simulink model "hvac"  (R2021b)
settings: Solver=FixedStepAuto  StartTime=0.0  StopTime=inf  FixedStep=.1  RelTol=1e-3  AbsTol=1e-6
InitFcn:
  | mpath = get_param(bdroot, 'FileName')
  | [path,name,ext]=fileparts(mpath)
  | path
  | addpath(path);
  | load('testData.mat')
StopFcn:
  | if isLogging
  |     outputJson = jsonencode(struct("simTime", output.simTime, "InsideTemp1", simOutput.InsideTemp1, "OutsideTemp1", simOutput.OutsideTemp1, "Heat1", simInput.Heat1, "Cool1", simInput.Cool1, ...
  |         "InsideTemp2", simOutput.InsideTemp2, "OutsideTemp2", simOutput.OutsideTemp2, "Heat2", simInput.Heat2, "Cool2", simInput.Cool2));
  |     fprintf(outputFile, "%s,", outputJson);
  |     fclose(outputFile);
  | end
model workspace (MATLAB code in the model file + MAT data in the model file):
  LWall = 0.2
  LWindow = 0.01
  M = 1778.36911446
  Mdot = 1
  PLC_IP_Address = 'localhost'
  RWall = 1.52148180317e-06
  RWindow = 5.93542260209e-07
  Req = 0.00153711229591
  THeater = 50
  TinIC = 20
  c = 1005.4
  cost = 2.5e-08
  densAir = 1.225
  htHouse = 4
  htWindows = 1
  kWall = 136.8
  kWindow = 2808
  lenHouse = 30
  numWindows = 6
  pitRoof = 0.698131700798
  r2d = 57.2957795131
  wallArea = 960.897659797
  widHouse = 10
  widWindows = 1
  windowArea = 6
  other statements: sldemo_househeat_data
undefined symbols (not defined in the file or in its folder): simInput
libraries: simulink_extras x4
PauseFcn:
  | if exist("fixedStepSize", "var") == 0
  |     fixedStepSize = simOutput.SimulationMetadata.ModelInfo.SolverInfo.FixedStepSize;
  | end
  | output.simTime = simOutput.SimulationMetadata.ModelInfo.StopTime - fixedStepSize;
  | output.InsideTemp1 = simOutput.InsideTemp1;
  | output.OutsideTemp1 = simOutput.OutsideTemp1;
  | output.InsideTemp2 = simOutput.InsideTemp2;
  | output.OutsideTemp2 = simOutput.OutsideTemp2;
ContinueFcn:
  | if isLogging
  |     outputJson = jsonencode(struct("simTime", output.simTime, "InsideTemp1", simOutput.InsideTemp1, "OutsideTemp1", simOutput.OutsideTemp1, "Heat1", simInput.Heat1, "Cool1", simInput.Cool1, ...
  |         "InsideTemp2", simOutput.InsideTemp2, "OutsideTemp2", simOutput.OutsideTemp2, "Heat2", simInput.Heat2, "Cool2", simInput.Cool2));
  |     fprintf(outputFile, "%s,", outputJson);
  | end
Description:
  | Thermal Model of a House
  | 
  | This demo illustrates how you can use Simulink(R) to create the thermal model of
  | a house. This system models the outdoor environment, the thermal
  | characteristics of the house, and the house heating system.
  | 
  | The sldemo_househeat_data.m file initializes data in the model workspace.
  | To make changes, you can edit the model workspace directly or edit the MATLAB(R) file
  | and re-load the model workspace.
  | 
  | To view the model workspace, select View > Model Explorer
  | from the Simulink editor.
  | 
  | Note: Time is given in units of hours
settings Model: PacingRate=100  Creator=The MathWorks, Inc.  LastModifiedBy=CCRE
settings SolverCC: AutoScaleAbsTol=off  AlgebraicLoopSolver=TrustRegion
settings DataIOCC: ExternalInput=[]  InitialState=[]  SaveFormat=Array  SaveOutput=off  SaveTime=off  SignalLoggingName=sldemo_househeat_output  ReturnWorkspaceOutputsName=simOutput
settings OptimizationCC: BlockReduction=off  BooleanDataType=off  ExpressionDepthLimit=2147483647  InitFltsAndDblsToZero=on  LifeSpan=inf  BufferReusableBoundary=off
settings DebuggingCC: SaveWithParameterizedLinksMsg=none  UnderspecifiedInitializationDetection=Classic  MergeDetectMultiDrivingBlocksExec=none  SignalResolutionControl=TryResolveAllWithWarning  MultiTaskDSMMsg=warning  MultiTaskCondExecSysMsg=none  IntegerOverflowMsg=none  FcnCallInpInsideContextMsg=warning  BusObjectLabelMismatch=none  StateNameClashWarn=warning  SFUnexpectedBacktrackingDiag=warning  SFNoUnconditionalDefaultTransitionDiag=warning  SFExecutionAtInitializationDiag=none  SFMachineParentedDataDiag=warning  IntegerSaturationMsg=none  ArithmeticOperatorsInVariantConditions=warning
settings HardwareCC: ProdBitPerPointer=32  ProdBitPerSizeT=32  ProdBitPerPtrDiffT=32  ProdLargestAtomicFloat=None  ProdIntDivRoundTo=Undefined  ProdEndianess=Unspecified  ProdWordSize=32  ProdHWDeviceType=32-bit Generic  TargetBitPerPointer=64  TargetBitPerSizeT=64  TargetBitPerPtrDiffT=64  TargetLongLongMode=on  TargetIntDivRoundTo=Zero  TargetEndianess=LittleEndian  TargetWordSize=64  TargetHWDeviceType=MATLAB Host  ProdEqTarget=off
settings ModelReferenceCC: PropagateSignalLabelsOutOfModel=off
settings SFSimCC: SimUseLocalCustomCode=off  CustomCodeUndefinedFunction=UseInterfaceOnly
settings RTWCC: PackageGeneratedCodeAndArtifacts=on  PackageName=HVAC  RTWUseLocalCustomCode=off
settings CodeAppCC: StateflowObjectComments=on
settings GRTTargetCC: TargetFcnLib=ansi_tfl_tmw.mat  TargetLangStandard=C89/C90 (ANSI)  CombineOutputUpdateFcns=off  GRTInterface=on
settings ConfigComp: CovMetricSettings=dw  CovSaveCumulativeToWorkspaceVar=on  CovSaveSingleToWorkspaceVar=on  CovExternalEMLEnable=off

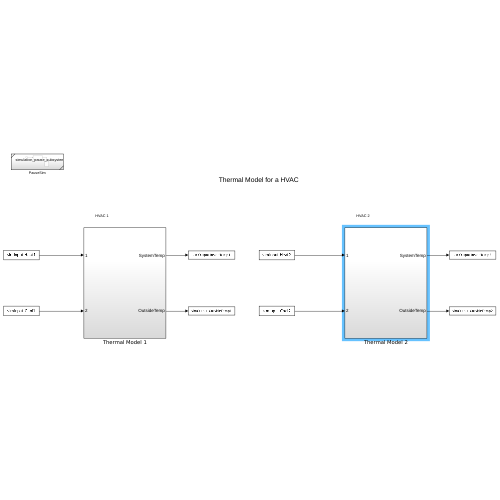
[thumbnail: Simulink's stored preview of the top-level diagram]
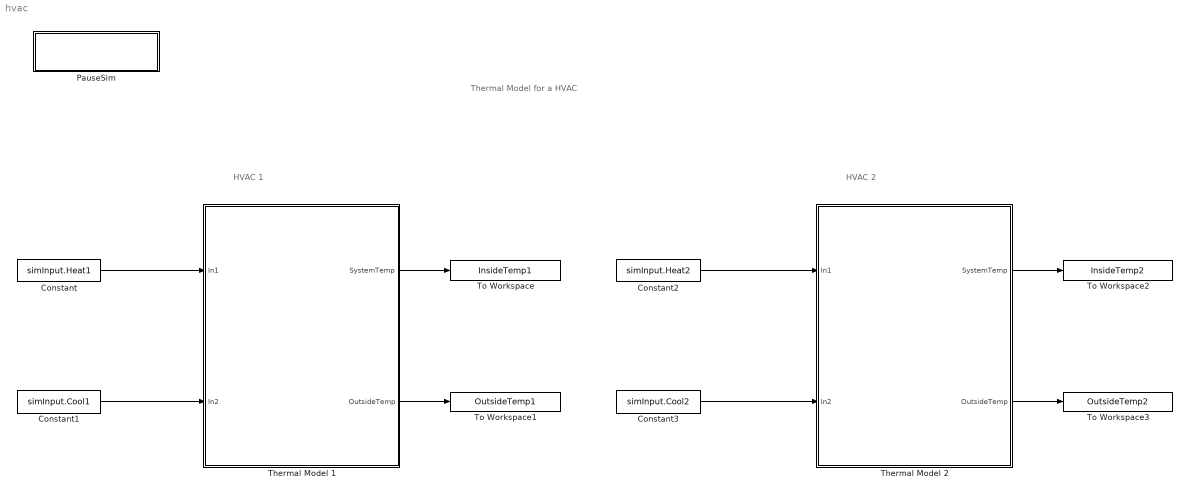
== system hvac ==
  note: HVAC 1
  note: Thermal Model for a HVAC
  note: HVAC 2
  Constant : Constant  Value=simInput.Heat1
  Constant1 : Constant  Value=simInput.Cool1
  Constant2 : Constant  Value=simInput.Heat2
  Constant3 : Constant  Value=simInput.Cool2
  PauseSim : Subsystem  ReferencedSubsystem=simulation_pause_subsystem
  Thermal Model 1 : Subsystem
  Thermal Model 2 : Subsystem
  To Workspace : ToWorkspace  VariableName=InsideTemp1  SampleTime=-1
      settings: MaxDataPoints=1  Save2DSignal=2-D array (concatenate along first dimension)
  To Workspace1 : ToWorkspace  VariableName=OutsideTemp1  SampleTime=-1
      settings: MaxDataPoints=1  Save2DSignal=2-D array (concatenate along first dimension)
  To Workspace2 : ToWorkspace  VariableName=InsideTemp2  SampleTime=-1
      settings: MaxDataPoints=1  Save2DSignal=2-D array (concatenate along first dimension)
  To Workspace3 : ToWorkspace  VariableName=OutsideTemp2  SampleTime=-1
      settings: MaxDataPoints=1  Save2DSignal=2-D array (concatenate along first dimension)
  wires:
  Thermal Model 1/1(SystemTemp) -> To Workspace/1
  Constant1/1 -> Thermal Model 1/2(In2)
  Thermal Model 1/2(OutsideTemp) -> To Workspace1/1
  Constant3/1 -> Thermal Model 2/2(In2)
  Constant/1 -> Thermal Model 1/1(In1)
  Constant2/1 -> Thermal Model 2/1(In1)
  Thermal Model 2/2(OutsideTemp) -> To Workspace3/1
  Thermal Model 2/1(SystemTemp) -> To Workspace2/1

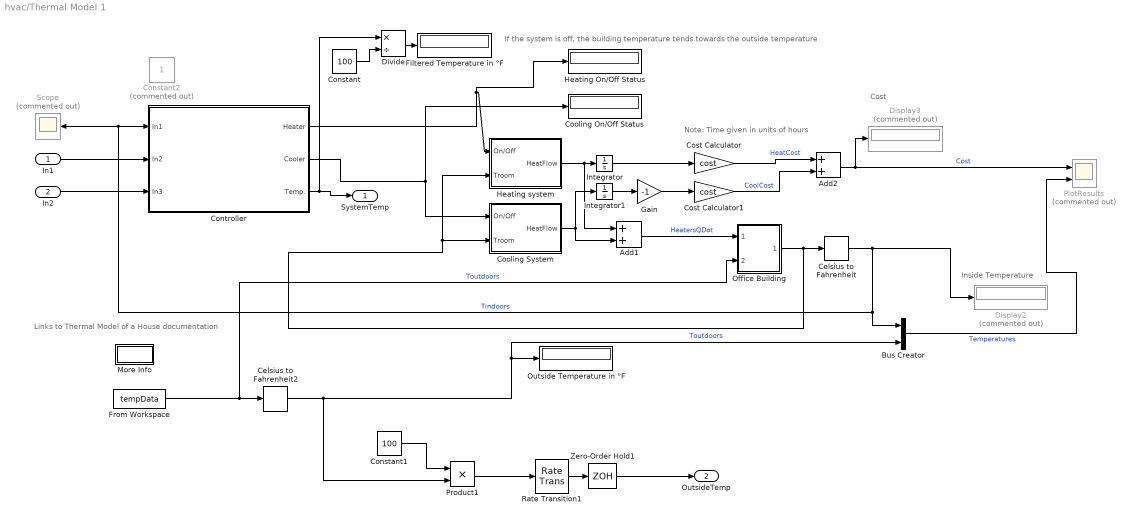
== system hvac/Thermal Model 1 ==
  note: If the system is off, the building temperature tends towards the outside temperature
  note: Links to Thermal Model of a House documentation
  note: Cost
  note: Inside Temperature
  note: Note: Time given in units of hours
  In1 : Inport
  In2 : Inport  Port=2
  Add1 : Sum
  Add2 : Sum
  Bus Creator : BusCreator  Inputs=2
  Celsius to Fahrenheit : simulink_extras/Transformations/Celsius to Fahrenheit
      settings: SourceProductBaseCode=SL
  Celsius to Fahrenheit2 : simulink_extras/Transformations/Celsius to Fahrenheit
      settings: SourceProductBaseCode=SL
  Constant : Constant  Value=100
  Constant1 : Constant  Value=100
  Constant2 : Constant  Commented=on
  Controller : Subsystem
  Cooling On/Off Status : Display
  Cooling System : Subsystem
  Cost Calculator : Gain  Gain=cost  SaturateOnIntegerOverflow=on  OutDataTypeStr=Inherit: Same as input  ParamDataTypeStr=Inherit: Same as input
  Cost Calculator1 : Gain  Gain=cost  SaturateOnIntegerOverflow=on  OutDataTypeStr=Inherit: Same as input  ParamDataTypeStr=Inherit: Same as input
  Display2 : Display  Commented=on
  Display3 : Display  Commented=on
  Divide : Product  Inputs=*/
  Filtered Temperature in °F : Display
  From Workspace : FromWorkspace  VariableName=tempData
  Gain : Gain  Gain=-1
  Heating On/Off Status : Display
  Heating system : Subsystem
  Integrator : Integrator
  Integrator1 : Integrator
  More Info : Subsystem
      settings: OpenFcn=showExample('simulink_general/sldemo_househeatExample')
      mask Display: disp('?')
  Office Building : Subsystem
      mask Display: image(fullfile('office-block-pic.jpg'))
  Outside Temperature in °F : Display
  PlotResults : Scope  Commented=on  NumInputPorts=2
  Product1 : Product
  Rate Transition1 : RateTransition
  Scope : Scope  Commented=on
  Zero-Order Hold1 : ZeroOrderHold  SampleTime=-1
  SystemTemp : Outport  VectorParamsAs1DForOutWhenUnconnected=off
  OutsideTemp : Outport  Port=2  VectorParamsAs1DForOutWhenUnconnected=off
  wires:
  From Workspace/1 -> Celsius to Fahrenheit2/1, Office Building/2(Outdoor Temp Tout)  "Toutdoors"
  Cost Calculator/1 -> Add2/1  "HeatCost"
  Integrator1/1 -> Gain/1
  Heating system/1(HeatFlow) -> Add1/1, Integrator/1
  Cooling System/1(HeatFlow) -> Add1/2, Integrator1/1
  Add2/1 -> PlotResults/1, Display3/1  "Cost"
  Add1/1 -> Office Building/1(Heater QDot In)  "HeatersQDot"
  Bus Creator/1 -> PlotResults/2  "Temperatures"
  Integrator/1 -> Cost Calculator/1
  Cost Calculator1/1 -> Add2/2  "CoolCost"
  Controller/2(Cooler) -> Cooling On/Off Status/1, Cooling System/1(On/Off)
  Gain/1 -> Cost Calculator1/1
  Controller/3(Temp.) -> Divide/1, SystemTemp/1
  Office Building/1(Room Temp Troom) -> Heating system/2(Troom), Cooling System/2(Troom), Celsius to Fahrenheit/1
  In1/1 -> Controller/2(In2)
  In2/1 -> Controller/3(In3)
  Celsius to Fahrenheit/1 -> Display2/1, Controller/1(In1), Scope/1, Bus Creator/1  "Tindoors"
  Constant/1 -> Divide/2
  Divide/1 -> Filtered Temperature in °F/1
  Rate Transition1/1 -> Zero-Order Hold1/1
  Constant1/1 -> Product1/1
  Celsius to Fahrenheit2/1 -> Product1/2, Bus Creator/2, Outside Temperature in °F/1  "Toutdoors"
  Controller/1(Heater) -> Heating On/Off Status/1, Heating system/1(On/Off)
  Product1/1 -> Rate Transition1/1
  Zero-Order Hold1/1 -> OutsideTemp/1

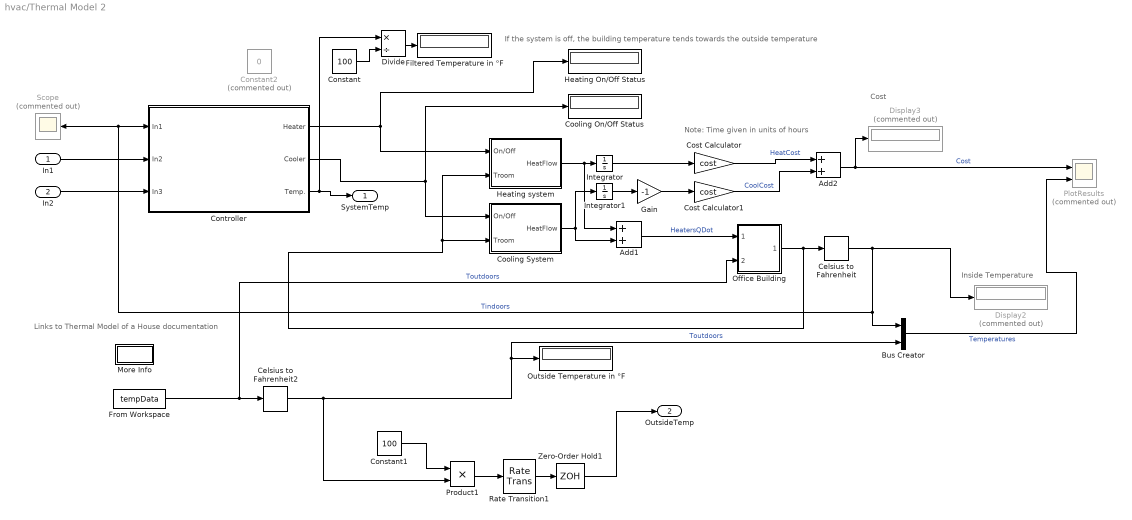
== system hvac/Thermal Model 2 ==
  note: If the system is off, the building temperature tends towards the outside temperature
  note: Links to Thermal Model of a House documentation
  note: Cost
  note: Inside Temperature
  note: Note: Time given in units of hours
  In1 : Inport
  In2 : Inport  Port=2
  Add1 : Sum
  Add2 : Sum
  Bus Creator : BusCreator  Inputs=2
  Celsius to Fahrenheit : simulink_extras/Transformations/Celsius to Fahrenheit
      settings: SourceProductBaseCode=SL
  Celsius to Fahrenheit2 : simulink_extras/Transformations/Celsius to Fahrenheit
      settings: SourceProductBaseCode=SL
  Constant : Constant  Value=100
  Constant1 : Constant  Value=100
  Constant2 : Constant  Commented=on  Value=0
  Controller : Subsystem
  Cooling On/Off Status : Display
  Cooling System : Subsystem
  Cost Calculator : Gain  Gain=cost  SaturateOnIntegerOverflow=on  OutDataTypeStr=Inherit: Same as input  ParamDataTypeStr=Inherit: Same as input
  Cost Calculator1 : Gain  Gain=cost  SaturateOnIntegerOverflow=on  OutDataTypeStr=Inherit: Same as input  ParamDataTypeStr=Inherit: Same as input
  Display2 : Display  Commented=on
  Display3 : Display  Commented=on
  Divide : Product  Inputs=*/
  Filtered Temperature in °F : Display
  From Workspace : FromWorkspace  VariableName=tempData
  Gain : Gain  Gain=-1
  Heating On/Off Status : Display
  Heating system : Subsystem
  Integrator : Integrator
  Integrator1 : Integrator
  More Info : Subsystem
      settings: OpenFcn=showExample('simulink_general/sldemo_househeatExample')
      mask Display: disp('?')
  Office Building : Subsystem
      mask Display: image(fullfile('office-block-pic.jpg'))
  Outside Temperature in °F : Display
  PlotResults : Scope  Commented=on  NumInputPorts=2
  Product1 : Product
  Rate Transition1 : RateTransition
  Scope : Scope  Commented=on
  Zero-Order Hold1 : ZeroOrderHold  SampleTime=-1
  SystemTemp : Outport  VectorParamsAs1DForOutWhenUnconnected=off
  OutsideTemp : Outport  Port=2  VectorParamsAs1DForOutWhenUnconnected=off
  wires:
  From Workspace/1 -> Celsius to Fahrenheit2/1, Office Building/2(Outdoor Temp Tout)  "Toutdoors"
  Cost Calculator/1 -> Add2/1  "HeatCost"
  Integrator1/1 -> Gain/1
  Heating system/1(HeatFlow) -> Add1/1, Integrator/1
  Cooling System/1(HeatFlow) -> Add1/2, Integrator1/1
  Add2/1 -> PlotResults/1, Display3/1  "Cost"
  Add1/1 -> Office Building/1(Heater QDot In)  "HeatersQDot"
  Bus Creator/1 -> PlotResults/2  "Temperatures"
  Integrator/1 -> Cost Calculator/1
  Cost Calculator1/1 -> Add2/2  "CoolCost"
  Controller/2(Cooler) -> Cooling On/Off Status/1, Cooling System/1(On/Off)
  Gain/1 -> Cost Calculator1/1
  Controller/3(Temp.) -> Divide/1, SystemTemp/1
  Office Building/1(Room Temp Troom) -> Heating system/2(Troom), Cooling System/2(Troom), Celsius to Fahrenheit/1
  In1/1 -> Controller/2(In2)
  In2/1 -> Controller/3(In3)
  Celsius to Fahrenheit/1 -> Display2/1, Controller/1(In1), Scope/1, Bus Creator/1  "Tindoors"
  Constant/1 -> Divide/2
  Divide/1 -> Filtered Temperature in °F/1
  Rate Transition1/1 -> Zero-Order Hold1/1
  Constant1/1 -> Product1/1
  Product1/1 -> Rate Transition1/1
  Celsius to Fahrenheit2/1 -> Product1/2, Bus Creator/2, Outside Temperature in °F/1  "Toutdoors"
  Zero-Order Hold1/1 -> OutsideTemp/1
  Controller/1(Heater) -> Heating On/Off Status/1, Heating system/1(On/Off)

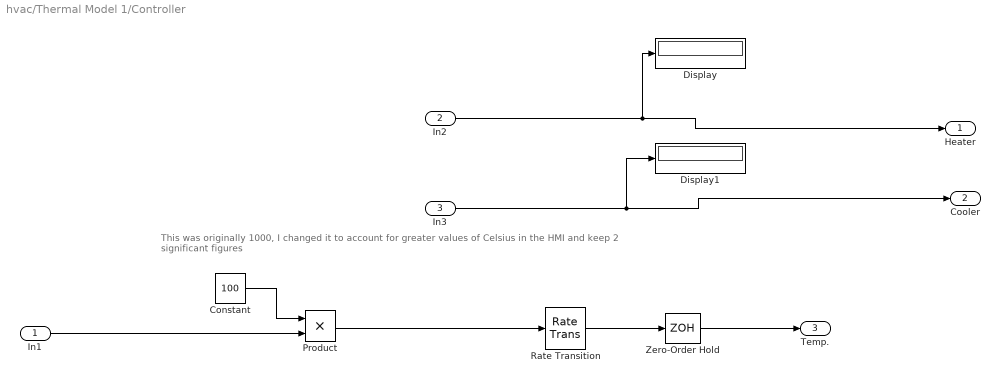
== system hvac/Thermal Model 1/Controller ==
  note: This was originally 1000,
      | I changed it to account for greater values of Celsius in the HMI and keep 2 significant figures
  In1 : Inport
  In2 : Inport  Port=2
  In3 : Inport  Port=3
  Constant : Constant  Value=100
  Display : Display
  Display1 : Display
  Product : Product
  Rate Transition : RateTransition
  Zero-Order Hold : ZeroOrderHold  SampleTime=-1
  Heater : Outport  VectorParamsAs1DForOutWhenUnconnected=off
  Cooler : Outport  Port=2  VectorParamsAs1DForOutWhenUnconnected=off
  Temp. : Outport  Port=3  VectorParamsAs1DForOutWhenUnconnected=off
  wires:
  Constant/1 -> Product/1
  In1/1 -> Product/2
  Rate Transition/1 -> Zero-Order Hold/1
  Product/1 -> Rate Transition/1
  Zero-Order Hold/1 -> Temp./1
  In2/1 -> Display/1, Heater/1
  In3/1 -> Display1/1, Cooler/1

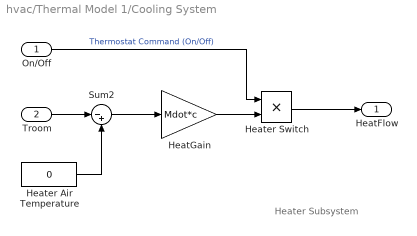
== system hvac/Thermal Model 1/Cooling System ==
  note: Heater Subsystem
  On/Off : Inport
  Troom : Inport  Port=2
  HeatGain : Gain  Gain=Mdot*c
  Heater Air Temperature : Constant  Value=0
  Heater Switch : Product  RndMeth=Zero
  Sum2 : Sum  Inputs=|-+
  HeatFlow : Outport  VectorParamsAs1DForOutWhenUnconnected=off
  wires:
  Heater Air Temperature/1 -> Sum2/2
  Troom/1 -> Sum2/1
  Sum2/1 -> HeatGain/1
  On/Off/1 -> Heater Switch/1  "Thermostat Command (On/Off)"
  HeatGain/1 -> Heater Switch/2
  Heater Switch/1 -> HeatFlow/1

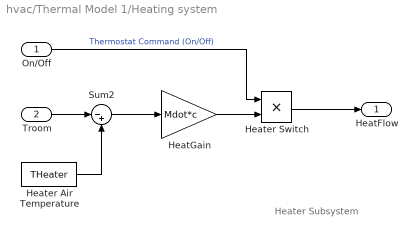
== system hvac/Thermal Model 1/Heating system ==
  note: Heater Subsystem
  On/Off : Inport
  Troom : Inport  Port=2
  HeatGain : Gain  Gain=Mdot*c
  Heater Air Temperature : Constant  Value=THeater
  Heater Switch : Product  RndMeth=Zero
  Sum2 : Sum  Inputs=|-+
  HeatFlow : Outport  VectorParamsAs1DForOutWhenUnconnected=off
  wires:
  Heater Air Temperature/1 -> Sum2/2
  Troom/1 -> Sum2/1
  Sum2/1 -> HeatGain/1
  On/Off/1 -> Heater Switch/1  "Thermostat Command (On/Off)"
  HeatGain/1 -> Heater Switch/2
  Heater Switch/1 -> HeatFlow/1

== system hvac/Thermal Model 1/More Info ==

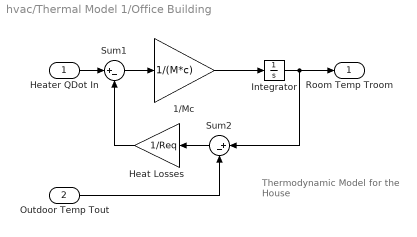
== system hvac/Thermal Model 1/Office Building ==
  note: Thermodynamic Model
      | for the House
  Heater QDot In : Inport
  Outdoor Temp Tout : Inport  Port=2
  1/Mc : Gain  Gain=1/(M*c)  SaturateOnIntegerOverflow=on  OutDataTypeStr=Inherit: Same as input  ParamDataTypeStr=Inherit: Same as input
  Heat Losses : Gain  Gain=1/Req  SaturateOnIntegerOverflow=on  OutDataTypeStr=Inherit: Same as input  ParamDataTypeStr=Inherit: Same as input
  Integrator : Integrator  InitialCondition=TinIC
  Sum1 : Sum  Inputs=|+-  InputSameDT=on  SaturateOnIntegerOverflow=on  OutDataTypeStr=Inherit: Same as first input
  Sum2 : Sum  Inputs=|+-  InputSameDT=on  SaturateOnIntegerOverflow=on  OutDataTypeStr=Inherit: Same as first input
  Room Temp Troom : Outport  InitialOutput=0  VectorParamsAs1DForOutWhenUnconnected=off
  wires:
  Outdoor Temp Tout/1 -> Sum2/2
  Heater QDot In/1 -> Sum1/1
  Sum1/1 -> 1/Mc/1
  Sum2/1 -> Heat Losses/1
  Heat Losses/1 -> Sum1/2
  1/Mc/1 -> Integrator/1
  Integrator/1 -> Sum2/1, Room Temp Troom/1

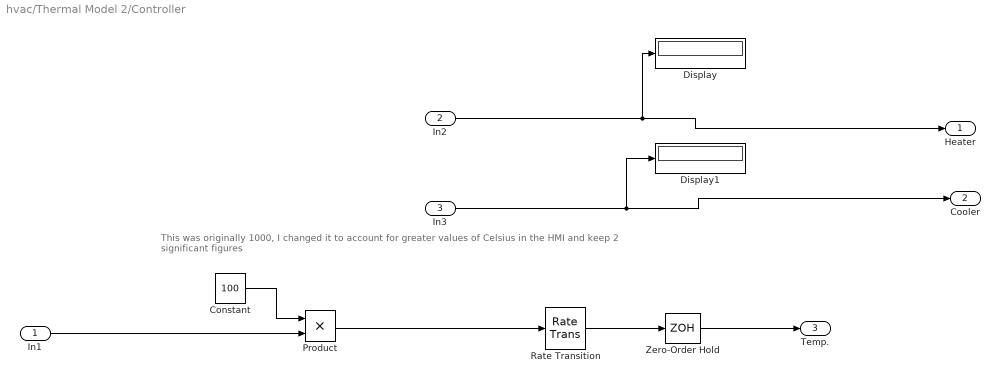
== system hvac/Thermal Model 2/Controller ==
  note: This was originally 1000,
      | I changed it to account for greater values of Celsius in the HMI and keep 2 significant figures
  In1 : Inport
  In2 : Inport  Port=2
  In3 : Inport  Port=3
  Constant : Constant  Value=100
  Display : Display
  Display1 : Display
  Product : Product
  Rate Transition : RateTransition
  Zero-Order Hold : ZeroOrderHold  SampleTime=-1
  Heater : Outport  VectorParamsAs1DForOutWhenUnconnected=off
  Cooler : Outport  Port=2  VectorParamsAs1DForOutWhenUnconnected=off
  Temp. : Outport  Port=3  VectorParamsAs1DForOutWhenUnconnected=off
  wires:
  Constant/1 -> Product/1
  In1/1 -> Product/2
  Rate Transition/1 -> Zero-Order Hold/1
  Product/1 -> Rate Transition/1
  Zero-Order Hold/1 -> Temp./1
  In2/1 -> Display/1, Heater/1
  In3/1 -> Display1/1, Cooler/1

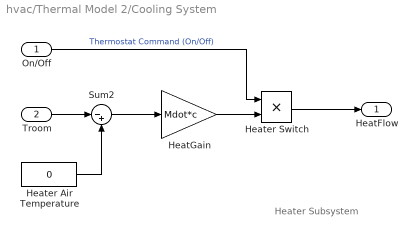
== system hvac/Thermal Model 2/Cooling System ==
  note: Heater Subsystem
  On/Off : Inport
  Troom : Inport  Port=2
  HeatGain : Gain  Gain=Mdot*c
  Heater Air Temperature : Constant  Value=0
  Heater Switch : Product  RndMeth=Zero
  Sum2 : Sum  Inputs=|-+
  HeatFlow : Outport  VectorParamsAs1DForOutWhenUnconnected=off
  wires:
  Heater Air Temperature/1 -> Sum2/2
  Troom/1 -> Sum2/1
  Sum2/1 -> HeatGain/1
  On/Off/1 -> Heater Switch/1  "Thermostat Command (On/Off)"
  HeatGain/1 -> Heater Switch/2
  Heater Switch/1 -> HeatFlow/1

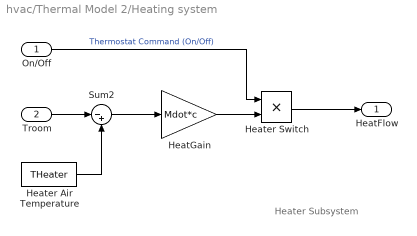
== system hvac/Thermal Model 2/Heating system ==
  note: Heater Subsystem
  On/Off : Inport
  Troom : Inport  Port=2
  HeatGain : Gain  Gain=Mdot*c
  Heater Air Temperature : Constant  Value=THeater
  Heater Switch : Product  RndMeth=Zero
  Sum2 : Sum  Inputs=|-+
  HeatFlow : Outport  VectorParamsAs1DForOutWhenUnconnected=off
  wires:
  Heater Air Temperature/1 -> Sum2/2
  Troom/1 -> Sum2/1
  Sum2/1 -> HeatGain/1
  On/Off/1 -> Heater Switch/1  "Thermostat Command (On/Off)"
  HeatGain/1 -> Heater Switch/2
  Heater Switch/1 -> HeatFlow/1

== system hvac/Thermal Model 2/More Info ==

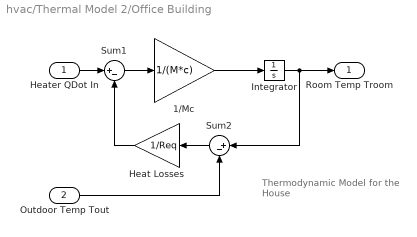
== system hvac/Thermal Model 2/Office Building ==
  note: Thermodynamic Model
      | for the House
  Heater QDot In : Inport
  Outdoor Temp Tout : Inport  Port=2
  1/Mc : Gain  Gain=1/(M*c)  SaturateOnIntegerOverflow=on  OutDataTypeStr=Inherit: Same as input  ParamDataTypeStr=Inherit: Same as input
  Heat Losses : Gain  Gain=1/Req  SaturateOnIntegerOverflow=on  OutDataTypeStr=Inherit: Same as input  ParamDataTypeStr=Inherit: Same as input
  Integrator : Integrator  InitialCondition=TinIC
  Sum1 : Sum  Inputs=|+-  InputSameDT=on  SaturateOnIntegerOverflow=on  OutDataTypeStr=Inherit: Same as first input
  Sum2 : Sum  Inputs=|+-  InputSameDT=on  SaturateOnIntegerOverflow=on  OutDataTypeStr=Inherit: Same as first input
  Room Temp Troom : Outport  InitialOutput=0  VectorParamsAs1DForOutWhenUnconnected=off
  wires:
  Outdoor Temp Tout/1 -> Sum2/2
  Heater QDot In/1 -> Sum1/1
  Sum1/1 -> 1/Mc/1
  Sum2/1 -> Heat Losses/1
  Heat Losses/1 -> Sum1/2
  1/Mc/1 -> Integrator/1
  Integrator/1 -> Sum2/1, Room Temp Troom/1
